simulink library "DDElib"  (Simulink 2.20)

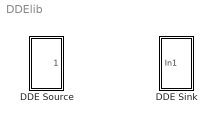
== system DDElib ==
  DDE Sink : Subsystem  mask(DDE Sink){service='excel', topic='test.xls', item='r1c1'}
      mask prompts: service "DDE Service:"; topic "DDE Topic:"; item "DDE Item:"
      mask Display: disp('DDE')
  DDE Source : Subsystem  mask(DDE Sink){service='excel', topic='test.xls', item='r1c1'}
      mask prompts: service "DDE Service:"; topic "DDE Topic:"; item "DDE Item:"
      mask Display: disp('DDE')

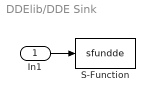
== system DDElib/DDE Sink ==
  In1 : Inport  Port=1  PortWidth=-1  SampleTime=-1
  S-Function : S-Function  FunctionName=sfundde  Parameters=service,topic,item  PortCounts=[]  SFunctionModules=''
  wires:
  In1/1 -> S-Function/1

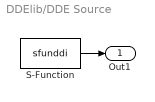
== system DDElib/DDE Source ==
  S-Function : S-Function  FunctionName=sfunddi  Parameters=service,topic,item  PortCounts=[]  SFunctionModules=''
  Out1 : Outport  Port=1
  wires:
  S-Function/1 -> Out1/1
